simulink model "Lab10Simple"  (R2017a)
settings: Solver=VariableStepAuto  StartTime=0.0  StopTime=0.5  MaxStep=0.001000001  MinStep=0.001  RelTol=1e-6
undefined symbols (not defined in the file): ip, K, Ka, Kf, Kw, Mcm, T_M, U
settings Model: Creator=User  LastModifiedBy=User

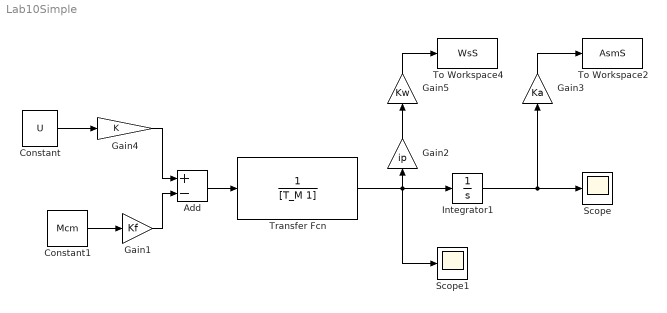
== system Lab10Simple ==
  Add : Sum  Inputs=+-
  Constant : Constant  Value=U
  Constant1 : Constant  Value=Mcm
  Gain1 : Gain  Gain=Kf
  Gain2 : Gain  Gain=ip
  Gain3 : Gain  Gain=Ka
  Gain4 : Gain  Gain=K
  Gain5 : Gain  Gain=Kw
  Integrator1 : Integrator
  Scope : Scope
  Scope1 : Scope
  To Workspace2 : ToWorkspace  VariableName=AsmS  SampleTime=-1
  To Workspace4 : ToWorkspace  VariableName=WsS  SampleTime=-1
  Transfer Fcn : TransferFcn  Denominator=[T_M 1]
  wires:
  Gain3/1 -> To Workspace2/1
  Transfer Fcn/1 -> Scope1/1, Gain2/1, Integrator1/1
  Add/1 -> Transfer Fcn/1
  Constant/1 -> Gain4/1
  Gain4/1 -> Add/1
  Constant1/1 -> Gain1/1
  Gain1/1 -> Add/2
  Gain2/1 -> Gain5/1
  Gain5/1 -> To Workspace4/1
  Integrator1/1 -> Gain3/1, Scope/1
